simulink model "im_foc_models_decouple"  (R2022b)
settings: Solver=VariableStepAuto  StartTime=0.0  StopTime=1  FixedStep=0.001  RelTol=1e-3
undefined symbols (not defined in the file): B, c, J, k, K1, K2, K3, K4, K5, K6, Lm, Lr, pole
libraries: slpidlib x5
settings Model: Creator=jack  LastModifiedBy=jackyeh

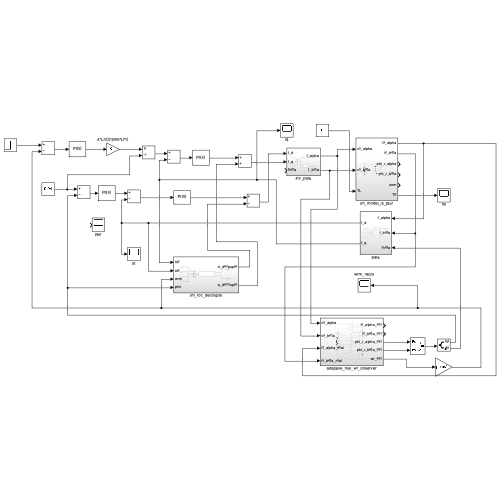
[thumbnail: Simulink's stored preview of the top-level diagram]
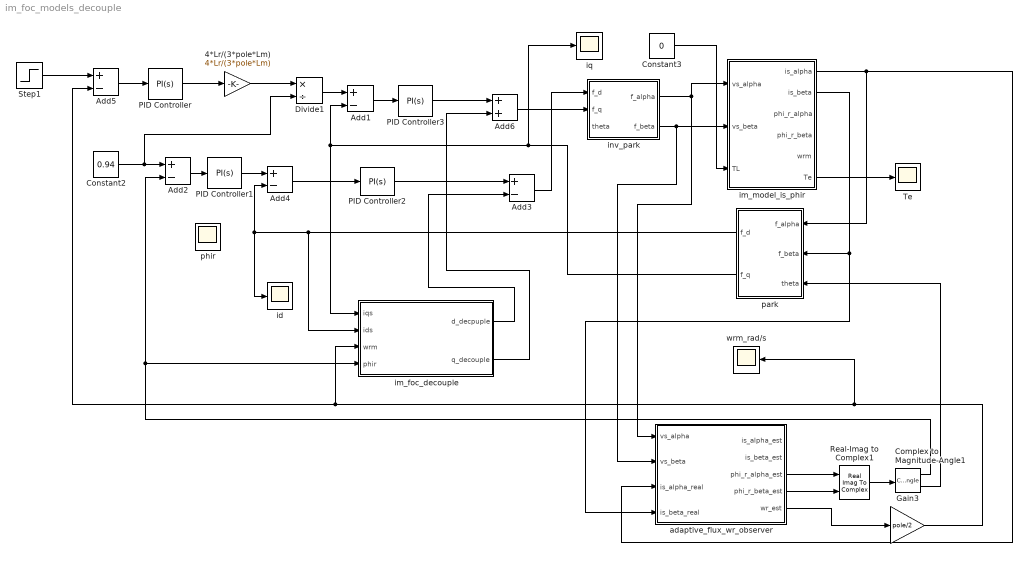
== system im_foc_models_decouple ==
  4*Lr/(3*pole*Lm) : Gain  Gain=4*Lr/(3*pole*Lm)
  Add{1..5} (5 alike) : Sum  Inputs=+-
  Add6 : Sum
  Complex to Magnitude-Angle1 : ComplexToMagnitudeAngle
  Constant2 : Constant  Value=0.94
  Constant3 : Constant  Value=0
  Divide1 : Product  Inputs=*/
  Gain3 : Gain  Gain=pole/2
  PID Controller : slpidlib/PID Controller  Controller=PI  Form=Parallel  TimeDomain=Continuous-time  UseExternalTs=off  SampleTime=-1  IntegratorMethod=Forward Euler  FilterMethod=Forward Euler  ControllerParametersSource=internal  P=1.65  I=0.41  UseKiTs=off  D=0  N=100  UseFilter=on  TunerSelectOption=Transfer Function Based (PID Tuner App)  InitialConditionSource=internal  InitialConditionForIntegrator=0  InitialConditionForFilter=0  DifferentiatorICPrevScaledInput=0  ExternalReset=none  TrackingMode=off  Kt=1  LimitOutput=off  SatLimitsSource=internal  UpperSaturationLimit=inf  LowerSaturationLimit=-inf  LinearizeAsGain=on  AntiWindupMode=none  Kb=1  LimitIntegrator=off  UpperIntegratorSaturationLimit=inf  LowerIntegratorSaturationLimit=-inf  POutMin=[]  POutMax=[]  IOutMin=[]  IOutMax=[]  DOutMin=[]  DOutMax=[]  NOutMin=[]  NOutMax=[]  SumOutMin=[]  SumOutMax=[]  SaturationOutMin=[]  SaturationOutMax=[]  PParamMin=[]  PParamMax=[]  IParamMin=[]  IParamMax=[]  DParamMin=[]  DParamMax=[]  NParamMin=[]  NParamMax=[]  KbParamMin=[]  KbParamMax=[]  KtParamMin=[]  KtParamMax=[]  KbOutMin=[]  KbOutMax=[]  KtOutMin=[]  KtOutMax=[]  IntegratorOutMin=[]  IntegratorOutMax=[]  FilterOutMin=[]  FilterOutMax=[]  SumI1OutMin=[]  SumI1OutMax=[]  SumI2OutMin=[]  SumI2OutMax=[]  SumI3OutMin=[]  SumI3OutMax=[]  SumI4OutMin=[]  SumI4OutMax=[]  SumDOutMin=[]  SumDOutMax=[]  DifferentiatorOutMin=[]  DifferentiatorOutMax=[]  FilterDiffOutCoefMin=[]  FilterDiffOutCoefMax=[]  ReciprocalOutMin=[]  ReciprocalOutMax=[]  SumDenOutMin=[]  SumDenOutMax=[]  SumNumOutMin=[]  SumNumOutMax=[]  DivideOutMin=[]  DivideOutMax=[]  UdiffTsProdOutMin=[]  UdiffTsProdOutMax=[]  NTsProdOutMin=[]  NTsProdOutMax=[]  UintegralTsProdOutMin=[]  UintegralTsProdOutMax=[]  UngainTsProdOutMin=[]  UngainTsProdOutMax=[]  ClampingZeroOutDataTypeStr=Inherit: Inherit via back propagation  ClampingZeroOutMin=[]  ClampingZeroOutMax=[]  FilterDenConstantOutDataTypeStr=Inherit: Inherit via back propagation  FilterDenConstantOutMin=[]  FilterDenConstantOutMax=[]  PCopyOutDataTypeStr=Inherit: Inherit via back propagation  PCopyOutMin=[]  PCopyOutMax=[]  NCopyOutDataTypeStr=Inherit: Inherit via back propagation  NCopyOutMin=[]  NCopyOutMax=[]  IntegratorContinuousStateAttributes=''  IntegratorStateMustResolveToSignalObject=off  IntegratorRTWStateStorageClass=Auto  FilterContinuousStateAttributes=''  FilterStateMustResolveToSignalObject=off  FilterRTWStateStorageClass=Auto  ParallelPVariant=InternalParameters  IdealPVariant=Disabled  IVariant=InternalParameters  DVariant=Disabled  IntegratorVariant=Continuous  SatVariant=Disabled  AWVariant=Passthrough  PCopyVariant=Disabled  TRVariant=Disabled  FdbkBlocksVariant=Forward  IdealPFdbkVariant=Disabled  SatFdbkVariant=Disabled  DerivativeFilterVariant=Disabled  NVariant=Disabled  NCopyVariant=Disabled_SignalSpec  FilterICVariant=Disabled  IntegratorICVariant=InternalICs  ExternalResetVariant=Disabled  TRSumVariant=Passthrough  SumFdbkVariant=Disabled  SumVariant=Sum_PI  TsampFilterVariant=InternalTs  TsampNgainVariant=Passthrough  TsampIntegralVariant=Passthrough  ExternalSaturationOutDataTypeStr=Inherit: Same as second input
  PID Controller1 : slpidlib/PID Controller  Controller=PI  Form=Parallel  TimeDomain=Continuous-time  UseExternalTs=off  SampleTime=-1  IntegratorMethod=Forward Euler  FilterMethod=Forward Euler  ControllerParametersSource=internal  P=86.38  I=609.76  UseKiTs=off  D=0  N=100  UseFilter=on  TunerSelectOption=Transfer Function Based (PID Tuner App)  InitialConditionSource=internal  InitialConditionForIntegrator=0  InitialConditionForFilter=0  DifferentiatorICPrevScaledInput=0  ExternalReset=none  TrackingMode=off  Kt=1  LimitOutput=off  SatLimitsSource=internal  UpperSaturationLimit=inf  LowerSaturationLimit=-inf  LinearizeAsGain=on  AntiWindupMode=none  Kb=1  LimitIntegrator=off  UpperIntegratorSaturationLimit=inf  LowerIntegratorSaturationLimit=-inf  POutMin=[]  POutMax=[]  IOutMin=[]  IOutMax=[]  DOutMin=[]  DOutMax=[]  NOutMin=[]  NOutMax=[]  SumOutMin=[]  SumOutMax=[]  SaturationOutMin=[]  SaturationOutMax=[]  PParamMin=[]  PParamMax=[]  IParamMin=[]  IParamMax=[]  DParamMin=[]  DParamMax=[]  NParamMin=[]  NParamMax=[]  KbParamMin=[]  KbParamMax=[]  KtParamMin=[]  KtParamMax=[]  KbOutMin=[]  KbOutMax=[]  KtOutMin=[]  KtOutMax=[]  IntegratorOutMin=[]  IntegratorOutMax=[]  FilterOutMin=[]  FilterOutMax=[]  SumI1OutMin=[]  SumI1OutMax=[]  SumI2OutMin=[]  SumI2OutMax=[]  SumI3OutMin=[]  SumI3OutMax=[]  SumI4OutMin=[]  SumI4OutMax=[]  SumDOutMin=[]  SumDOutMax=[]  DifferentiatorOutMin=[]  DifferentiatorOutMax=[]  FilterDiffOutCoefMin=[]  FilterDiffOutCoefMax=[]  ReciprocalOutMin=[]  ReciprocalOutMax=[]  SumDenOutMin=[]  SumDenOutMax=[]  SumNumOutMin=[]  SumNumOutMax=[]  DivideOutMin=[]  DivideOutMax=[]  UdiffTsProdOutMin=[]  UdiffTsProdOutMax=[]  NTsProdOutMin=[]  NTsProdOutMax=[]  UintegralTsProdOutMin=[]  UintegralTsProdOutMax=[]  UngainTsProdOutMin=[]  UngainTsProdOutMax=[]  ClampingZeroOutDataTypeStr=Inherit: Inherit via back propagation  ClampingZeroOutMin=[]  ClampingZeroOutMax=[]  FilterDenConstantOutDataTypeStr=Inherit: Inherit via back propagation  FilterDenConstantOutMin=[]  FilterDenConstantOutMax=[]  PCopyOutDataTypeStr=Inherit: Inherit via back propagation  PCopyOutMin=[]  PCopyOutMax=[]  NCopyOutDataTypeStr=Inherit: Inherit via back propagation  NCopyOutMin=[]  NCopyOutMax=[]  IntegratorContinuousStateAttributes=''  IntegratorStateMustResolveToSignalObject=off  IntegratorRTWStateStorageClass=Auto  FilterContinuousStateAttributes=''  FilterStateMustResolveToSignalObject=off  FilterRTWStateStorageClass=Auto  ParallelPVariant=InternalParameters  IdealPVariant=Disabled  IVariant=InternalParameters  DVariant=Disabled  IntegratorVariant=Continuous  SatVariant=Disabled  AWVariant=Passthrough  PCopyVariant=Disabled  TRVariant=Disabled  FdbkBlocksVariant=Forward  IdealPFdbkVariant=Disabled  SatFdbkVariant=Disabled  DerivativeFilterVariant=Disabled  NVariant=Disabled  NCopyVariant=Disabled_SignalSpec  FilterICVariant=Disabled  IntegratorICVariant=InternalICs  ExternalResetVariant=Disabled  TRSumVariant=Passthrough  SumFdbkVariant=Disabled  SumVariant=Sum_PI  TsampFilterVariant=InternalTs  TsampNgainVariant=Passthrough  TsampIntegralVariant=Passthrough  ExternalSaturationOutDataTypeStr=Inherit: Same as second input
  PID Controller2 : slpidlib/PID Controller  Controller=PI  Form=Parallel  TimeDomain=Continuous-time  UseExternalTs=off  SampleTime=-1  IntegratorMethod=Forward Euler  FilterMethod=Forward Euler  ControllerParametersSource=internal  P=2.95  I=679.2  UseKiTs=off  D=0  N=100  UseFilter=on  TunerSelectOption=Transfer Function Based (PID Tuner App)  InitialConditionSource=internal  InitialConditionForIntegrator=0  InitialConditionForFilter=0  DifferentiatorICPrevScaledInput=0  ExternalReset=none  TrackingMode=off  Kt=1  LimitOutput=off  SatLimitsSource=internal  UpperSaturationLimit=inf  LowerSaturationLimit=-inf  LinearizeAsGain=on  AntiWindupMode=none  Kb=1  LimitIntegrator=off  UpperIntegratorSaturationLimit=inf  LowerIntegratorSaturationLimit=-inf  POutMin=[]  POutMax=[]  IOutMin=[]  IOutMax=[]  DOutMin=[]  DOutMax=[]  NOutMin=[]  NOutMax=[]  SumOutMin=[]  SumOutMax=[]  SaturationOutMin=[]  SaturationOutMax=[]  PParamMin=[]  PParamMax=[]  IParamMin=[]  IParamMax=[]  DParamMin=[]  DParamMax=[]  NParamMin=[]  NParamMax=[]  KbParamMin=[]  KbParamMax=[]  KtParamMin=[]  KtParamMax=[]  KbOutMin=[]  KbOutMax=[]  KtOutMin=[]  KtOutMax=[]  IntegratorOutMin=[]  IntegratorOutMax=[]  FilterOutMin=[]  FilterOutMax=[]  SumI1OutMin=[]  SumI1OutMax=[]  SumI2OutMin=[]  SumI2OutMax=[]  SumI3OutMin=[]  SumI3OutMax=[]  SumI4OutMin=[]  SumI4OutMax=[]  SumDOutMin=[]  SumDOutMax=[]  DifferentiatorOutMin=[]  DifferentiatorOutMax=[]  FilterDiffOutCoefMin=[]  FilterDiffOutCoefMax=[]  ReciprocalOutMin=[]  ReciprocalOutMax=[]  SumDenOutMin=[]  SumDenOutMax=[]  SumNumOutMin=[]  SumNumOutMax=[]  DivideOutMin=[]  DivideOutMax=[]  UdiffTsProdOutMin=[]  UdiffTsProdOutMax=[]  NTsProdOutMin=[]  NTsProdOutMax=[]  UintegralTsProdOutMin=[]  UintegralTsProdOutMax=[]  UngainTsProdOutMin=[]  UngainTsProdOutMax=[]  ClampingZeroOutDataTypeStr=Inherit: Inherit via back propagation  ClampingZeroOutMin=[]  ClampingZeroOutMax=[]  FilterDenConstantOutDataTypeStr=Inherit: Inherit via back propagation  FilterDenConstantOutMin=[]  FilterDenConstantOutMax=[]  PCopyOutDataTypeStr=Inherit: Inherit via back propagation  PCopyOutMin=[]  PCopyOutMax=[]  NCopyOutDataTypeStr=Inherit: Inherit via back propagation  NCopyOutMin=[]  NCopyOutMax=[]  IntegratorContinuousStateAttributes=''  IntegratorStateMustResolveToSignalObject=off  IntegratorRTWStateStorageClass=Auto  FilterContinuousStateAttributes=''  FilterStateMustResolveToSignalObject=off  FilterRTWStateStorageClass=Auto  ParallelPVariant=InternalParameters  IdealPVariant=Disabled  IVariant=InternalParameters  DVariant=Disabled  IntegratorVariant=Continuous  SatVariant=Disabled  AWVariant=Passthrough  PCopyVariant=Disabled  TRVariant=Disabled  FdbkBlocksVariant=Forward  IdealPFdbkVariant=Disabled  SatFdbkVariant=Disabled  DerivativeFilterVariant=Disabled  NVariant=Disabled  NCopyVariant=Disabled_SignalSpec  FilterICVariant=Disabled  IntegratorICVariant=InternalICs  ExternalResetVariant=Disabled  TRSumVariant=Passthrough  SumFdbkVariant=Disabled  SumVariant=Sum_PI  TsampFilterVariant=InternalTs  TsampNgainVariant=Passthrough  TsampIntegralVariant=Passthrough  ExternalSaturationOutDataTypeStr=Inherit: Same as second input
  PID Controller3 : slpidlib/PID Controller  Controller=PI  Form=Parallel  TimeDomain=Continuous-time  UseExternalTs=off  SampleTime=-1  IntegratorMethod=Forward Euler  FilterMethod=Forward Euler  ControllerParametersSource=internal  P=2.95  I=400  UseKiTs=off  D=0  N=100  UseFilter=on  TunerSelectOption=Transfer Function Based (PID Tuner App)  InitialConditionSource=internal  InitialConditionForIntegrator=0  InitialConditionForFilter=0  DifferentiatorICPrevScaledInput=0  ExternalReset=none  TrackingMode=off  Kt=1  LimitOutput=off  SatLimitsSource=internal  UpperSaturationLimit=inf  LowerSaturationLimit=-inf  LinearizeAsGain=on  AntiWindupMode=none  Kb=1  LimitIntegrator=off  UpperIntegratorSaturationLimit=inf  LowerIntegratorSaturationLimit=-inf  POutMin=[]  POutMax=[]  IOutMin=[]  IOutMax=[]  DOutMin=[]  DOutMax=[]  NOutMin=[]  NOutMax=[]  SumOutMin=[]  SumOutMax=[]  SaturationOutMin=[]  SaturationOutMax=[]  PParamMin=[]  PParamMax=[]  IParamMin=[]  IParamMax=[]  DParamMin=[]  DParamMax=[]  NParamMin=[]  NParamMax=[]  KbParamMin=[]  KbParamMax=[]  KtParamMin=[]  KtParamMax=[]  KbOutMin=[]  KbOutMax=[]  KtOutMin=[]  KtOutMax=[]  IntegratorOutMin=[]  IntegratorOutMax=[]  FilterOutMin=[]  FilterOutMax=[]  SumI1OutMin=[]  SumI1OutMax=[]  SumI2OutMin=[]  SumI2OutMax=[]  SumI3OutMin=[]  SumI3OutMax=[]  SumI4OutMin=[]  SumI4OutMax=[]  SumDOutMin=[]  SumDOutMax=[]  DifferentiatorOutMin=[]  DifferentiatorOutMax=[]  FilterDiffOutCoefMin=[]  FilterDiffOutCoefMax=[]  ReciprocalOutMin=[]  ReciprocalOutMax=[]  SumDenOutMin=[]  SumDenOutMax=[]  SumNumOutMin=[]  SumNumOutMax=[]  DivideOutMin=[]  DivideOutMax=[]  UdiffTsProdOutMin=[]  UdiffTsProdOutMax=[]  NTsProdOutMin=[]  NTsProdOutMax=[]  UintegralTsProdOutMin=[]  UintegralTsProdOutMax=[]  UngainTsProdOutMin=[]  UngainTsProdOutMax=[]  ClampingZeroOutDataTypeStr=Inherit: Inherit via back propagation  ClampingZeroOutMin=[]  ClampingZeroOutMax=[]  FilterDenConstantOutDataTypeStr=Inherit: Inherit via back propagation  FilterDenConstantOutMin=[]  FilterDenConstantOutMax=[]  PCopyOutDataTypeStr=Inherit: Inherit via back propagation  PCopyOutMin=[]  PCopyOutMax=[]  NCopyOutDataTypeStr=Inherit: Inherit via back propagation  NCopyOutMin=[]  NCopyOutMax=[]  IntegratorContinuousStateAttributes=''  IntegratorStateMustResolveToSignalObject=off  IntegratorRTWStateStorageClass=Auto  FilterContinuousStateAttributes=''  FilterStateMustResolveToSignalObject=off  FilterRTWStateStorageClass=Auto  ParallelPVariant=InternalParameters  IdealPVariant=Disabled  IVariant=InternalParameters  DVariant=Disabled  IntegratorVariant=Continuous  SatVariant=Disabled  AWVariant=Passthrough  PCopyVariant=Disabled  TRVariant=Disabled  FdbkBlocksVariant=Forward  IdealPFdbkVariant=Disabled  SatFdbkVariant=Disabled  DerivativeFilterVariant=Disabled  NVariant=Disabled  NCopyVariant=Disabled_SignalSpec  FilterICVariant=Disabled  IntegratorICVariant=InternalICs  ExternalResetVariant=Disabled  TRSumVariant=Passthrough  SumFdbkVariant=Disabled  SumVariant=Sum_PI  TsampFilterVariant=InternalTs  TsampNgainVariant=Passthrough  TsampIntegralVariant=Passthrough  ExternalSaturationOutDataTypeStr=Inherit: Same as second input
  Real-Imag to Complex1 : RealImagToComplex
  Step1 : Step  Time=0  After=100  SampleTime=0
  Te : Scope
  adaptive_flux_wr_observer : Subsystem
  id : Scope
  im_foc_decouple : Subsystem
  im_model_is_phir : Subsystem
  inv_park : Subsystem
  iq : Scope
  park : Subsystem
  phir : Scope
  wrm_rad/s : Scope
  wires:
  PID Controller/1 -> 4*Lr/(3*pole*Lm)/1
  4*Lr/(3*pole*Lm)/1 -> Divide1/1
  Constant2/1 -> Divide1/2, Add2/1
  Divide1/1 -> Add1/1
  Add1/1 -> PID Controller3/1
  Add2/1 -> PID Controller1/1
  PID Controller1/1 -> Add4/1
  Add4/1 -> PID Controller2/1
  Add5/1 -> PID Controller/1
  Add6/1 -> inv_park/2(f_q)
  inv_park/1(f_alpha) -> im_model_is_phir/1(vs_alpha), adaptive_flux_wr_observer/1(vs_alpha)
  inv_park/2(f_beta) -> im_model_is_phir/2(vs_beta), adaptive_flux_wr_observer/2(vs_beta)
  Constant3/1 -> im_model_is_phir/3(TL)
  im_model_is_phir/1(is_alpha) -> adaptive_flux_wr_observer/3(is_alpha_real), park/1(f_alpha)
  im_model_is_phir/2(is_beta) -> adaptive_flux_wr_observer/4(is_beta_real), park/2(f_beta)
  park/2(f_q) -> im_foc_decouple/1(iqs), Add1/2, iq/1
  park/1(f_d) -> im_foc_decouple/2(ids), Add4/2, id/1
  Add3/1 -> inv_park/1(f_d)
  im_model_is_phir/6(Te) -> Te/1
  PID Controller2/1 -> Add3/1
  im_foc_decouple/1(d_decpuple) -> Add3/2
  PID Controller3/1 -> Add6/1
  im_foc_decouple/2(q_decouple) -> Add6/2
  Step1/1 -> Add5/1
  adaptive_flux_wr_observer/3(phi_r_alpha_est) -> Real-Imag to Complex1/1
  adaptive_flux_wr_observer/4(phi_r_beta_est) -> Real-Imag to Complex1/2
  Real-Imag to Complex1/1 -> Complex to Magnitude-Angle1/1
  Complex to Magnitude-Angle1/2 -> park/3(theta)
  Complex to Magnitude-Angle1/1 -> Add2/2, im_foc_decouple/4(phir)
  adaptive_flux_wr_observer/5(wr_est) -> Gain3/1
  Gain3/1 -> wrm_rad/s/1, im_foc_decouple/3(wrm), Add5/2

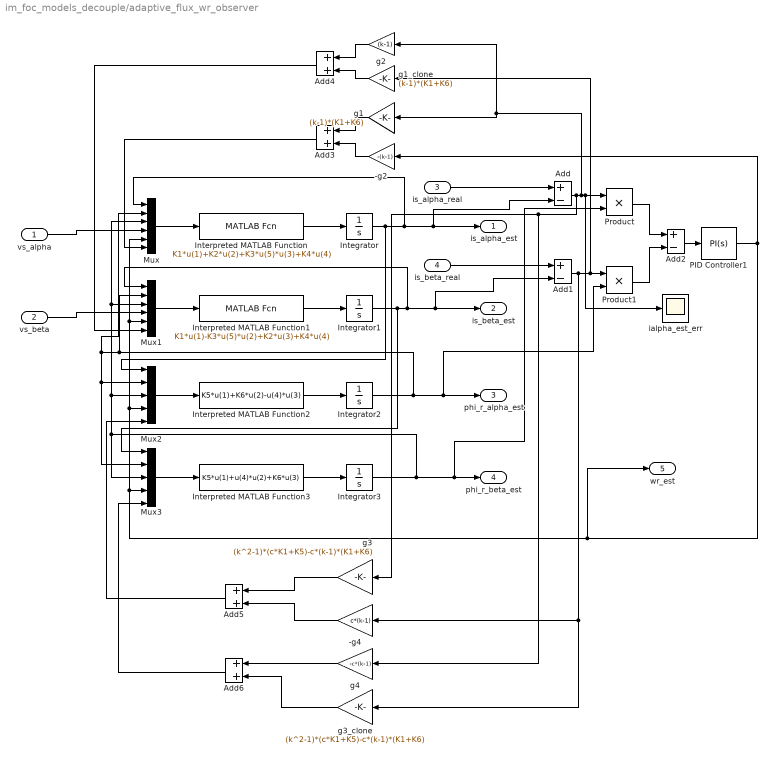
== system im_foc_models_decouple/adaptive_flux_wr_observer ==
  vs_alpha : Inport
  vs_beta : Inport  Port=2
  is_alpha_real : Inport  Port=3
  is_beta_real : Inport  Port=4
  -g2 : Gain  Gain=-(k-1)
  -g4 : Gain  Gain=c*(k-1)
  Add : Sum  Inputs=+-
  Add1 : Sum  Inputs=+-
  Add2 : Sum  Inputs=+-
  Add{3..6} (4 alike) : Sum
  Integrator{,1..3} (4 alike) : Integrator
  Interpreted MATLAB Function : MATLABFcn  MATLABFcn=K1*u(1)+K2*u(2)+K3*u(5)*u(3)+K4*u(4)
  Interpreted MATLAB Function1 : MATLABFcn  MATLABFcn=K1*u(1)-K3*u(5)*u(2)+K2*u(3)+K4*u(4)
  Interpreted MATLAB Function2 : MATLABFcn  MATLABFcn=K5*u(1)+K6*u(2)-u(4)*u(3)
  Interpreted MATLAB Function3 : MATLABFcn  MATLABFcn=K5*u(1)+u(4)*u(2)+K6*u(3)
  Mux : Mux  Inputs=6
  Mux1 : Mux  Inputs=6
  Mux2 : Mux  Inputs=5
  Mux3 : Mux  Inputs=5
  PID Controller1 : slpidlib/PID Controller  Controller=PI  Form=Parallel  TimeDomain=Continuous-time  UseExternalTs=off  SampleTime=-1  IntegratorMethod=Forward Euler  FilterMethod=Forward Euler  ControllerParametersSource=internal  P=542  I=3829  UseKiTs=off  D=0  N=100  UseFilter=on  TunerSelectOption=Transfer Function Based (PID Tuner App)  InitialConditionSource=internal  InitialConditionForIntegrator=0  InitialConditionForFilter=0  DifferentiatorICPrevScaledInput=0  ExternalReset=none  TrackingMode=off  Kt=1  LimitOutput=off  SatLimitsSource=internal  UpperSaturationLimit=inf  LowerSaturationLimit=-inf  LinearizeAsGain=on  AntiWindupMode=none  Kb=1  LimitIntegrator=off  UpperIntegratorSaturationLimit=inf  LowerIntegratorSaturationLimit=-inf  POutMin=[]  POutMax=[]  IOutMin=[]  IOutMax=[]  DOutMin=[]  DOutMax=[]  NOutMin=[]  NOutMax=[]  SumOutMin=[]  SumOutMax=[]  SaturationOutMin=[]  SaturationOutMax=[]  PParamMin=[]  PParamMax=[]  IParamMin=[]  IParamMax=[]  DParamMin=[]  DParamMax=[]  NParamMin=[]  NParamMax=[]  KbParamMin=[]  KbParamMax=[]  KtParamMin=[]  KtParamMax=[]  KbOutMin=[]  KbOutMax=[]  KtOutMin=[]  KtOutMax=[]  IntegratorOutMin=[]  IntegratorOutMax=[]  FilterOutMin=[]  FilterOutMax=[]  SumI1OutMin=[]  SumI1OutMax=[]  SumI2OutMin=[]  SumI2OutMax=[]  SumI3OutMin=[]  SumI3OutMax=[]  SumI4OutMin=[]  SumI4OutMax=[]  SumDOutMin=[]  SumDOutMax=[]  DifferentiatorOutMin=[]  DifferentiatorOutMax=[]  FilterDiffOutCoefMin=[]  FilterDiffOutCoefMax=[]  ReciprocalOutMin=[]  ReciprocalOutMax=[]  SumDenOutMin=[]  SumDenOutMax=[]  SumNumOutMin=[]  SumNumOutMax=[]  DivideOutMin=[]  DivideOutMax=[]  UdiffTsProdOutMin=[]  UdiffTsProdOutMax=[]  NTsProdOutMin=[]  NTsProdOutMax=[]  UintegralTsProdOutMin=[]  UintegralTsProdOutMax=[]  UngainTsProdOutMin=[]  UngainTsProdOutMax=[]  ClampingZeroOutDataTypeStr=Inherit: Inherit via back propagation  ClampingZeroOutMin=[]  ClampingZeroOutMax=[]  FilterDenConstantOutDataTypeStr=Inherit: Inherit via back propagation  FilterDenConstantOutMin=[]  FilterDenConstantOutMax=[]  PCopyOutDataTypeStr=Inherit: Inherit via back propagation  PCopyOutMin=[]  PCopyOutMax=[]  NCopyOutDataTypeStr=Inherit: Inherit via back propagation  NCopyOutMin=[]  NCopyOutMax=[]  IntegratorContinuousStateAttributes=''  IntegratorStateMustResolveToSignalObject=off  IntegratorRTWStateStorageClass=Auto  FilterContinuousStateAttributes=''  FilterStateMustResolveToSignalObject=off  FilterRTWStateStorageClass=Auto  ParallelPVariant=InternalParameters  IdealPVariant=Disabled  IVariant=InternalParameters  DVariant=Disabled  IntegratorVariant=Continuous  SatVariant=Disabled  AWVariant=Passthrough  PCopyVariant=Disabled  TRVariant=Disabled  FdbkBlocksVariant=Forward  IdealPFdbkVariant=Disabled  SatFdbkVariant=Disabled  DerivativeFilterVariant=Disabled  NVariant=Disabled  NCopyVariant=Disabled_SignalSpec  FilterICVariant=Disabled  IntegratorICVariant=InternalICs  ExternalResetVariant=Disabled  TRSumVariant=Passthrough  SumFdbkVariant=Disabled  SumVariant=Sum_PI  TsampFilterVariant=InternalTs  TsampNgainVariant=Passthrough  TsampIntegralVariant=Passthrough  ExternalSaturationOutDataTypeStr=Inherit: Same as second input
  Product : Product
  Product1 : Product
  g1 : Gain  Gain=(k-1)*(K1+K6)
  g1_clone : Gain  Gain=(k-1)*(K1+K6)
  g2 : Gain  Gain=(k-1)
  g3 : Gain  Gain=(k^2-1)*(c*K1+K5)-c*(k-1)*(K1+K6)
  g3_clone : Gain  Gain=(k^2-1)*(c*K1+K5)-c*(k-1)*(K1+K6)
  g4 : Gain  Gain=-c*(k-1)
  ialpha_est_err : Scope
  is_alpha_est : Outport
  is_beta_est : Outport  Port=2
  phi_r_alpha_est : Outport  Port=3
  phi_r_beta_est : Outport  Port=4
  wr_est : Outport  Port=5
  wires:
  Add3/1 -> Mux/6
  is_alpha_real/1 -> Add/1
  Mux1/1 -> Interpreted MATLAB Function1/1
  Interpreted MATLAB Function1/1 -> Integrator1/1
  Mux/1 -> Interpreted MATLAB Function/1
  Product1/1 -> Add2/2
  Integrator3/1 -> phi_r_beta_est/1, Product/2, Mux3/3, Mux2/3, Mux/3, Mux1/3
  vs_beta/1 -> Mux1/4
  Add5/1 -> Mux2/5
  Add/1 -> g4/1, g3/1, g2/1, g1/1, ialpha_est_err/1, Product/1
  is_beta_real/1 -> Add1/1
  Add4/1 -> Mux1/6
  g3/1 -> Add5/1
  g1_clone/1 -> Add4/2
  Integrator/1 -> Mux2/1, is_alpha_est/1, Add/2, Mux/1
  g1/1 -> Add3/1
  Interpreted MATLAB Function3/1 -> Integrator3/1
  g4/1 -> Add6/1
  Interpreted MATLAB Function/1 -> Integrator/1
  vs_alpha/1 -> Mux/4
  Add2/1 -> PID Controller1/1
  PID Controller1/1 -> wr_est/1, Mux3/4, Mux2/4, Mux1/5, Mux/5, -g2/1
  -g4/1 -> Add5/2
  Mux3/1 -> Interpreted MATLAB Function3/1
  g2/1 -> Add4/1
  Add6/1 -> Mux3/5
  Interpreted MATLAB Function2/1 -> Integrator2/1
  Integrator2/1 -> phi_r_alpha_est/1, Product1/2, Mux1/2, Mux/2, Mux3/2, Mux2/2
  Mux2/1 -> Interpreted MATLAB Function2/1
  -g2/1 -> Add3/2
  Product/1 -> Add2/1
  Integrator1/1 -> Mux3/1, is_beta_est/1, Add1/2, Mux1/1
  Add1/1 -> -g4/1, g3_clone/1, g1_clone/1, Product1/1
  g3_clone/1 -> Add6/2

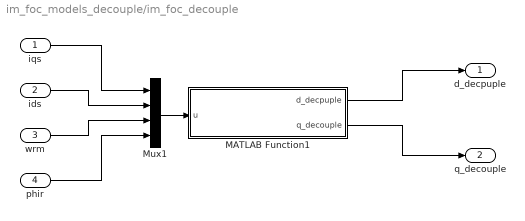
== system im_foc_models_decouple/im_foc_decouple ==
  iqs : Inport
  ids : Inport  Port=2
  wrm : Inport  Port=3
  phir : Inport  Port=4
  MATLAB Function1 : MATLAB Function  TreatAsAtomicUnit=on
  Mux1 : Mux
  d_decpuple : Outport
  q_decouple : Outport  Port=2
  wires:
  iqs/1 -> Mux1/1
  ids/1 -> Mux1/2
  wrm/1 -> Mux1/3
  Mux1/1 -> MATLAB Function1/1(u)
  MATLAB Function1/1(d_decpuple) -> d_decpuple/1
  MATLAB Function1/2(q_decouple) -> q_decouple/1
  phir/1 -> Mux1/4

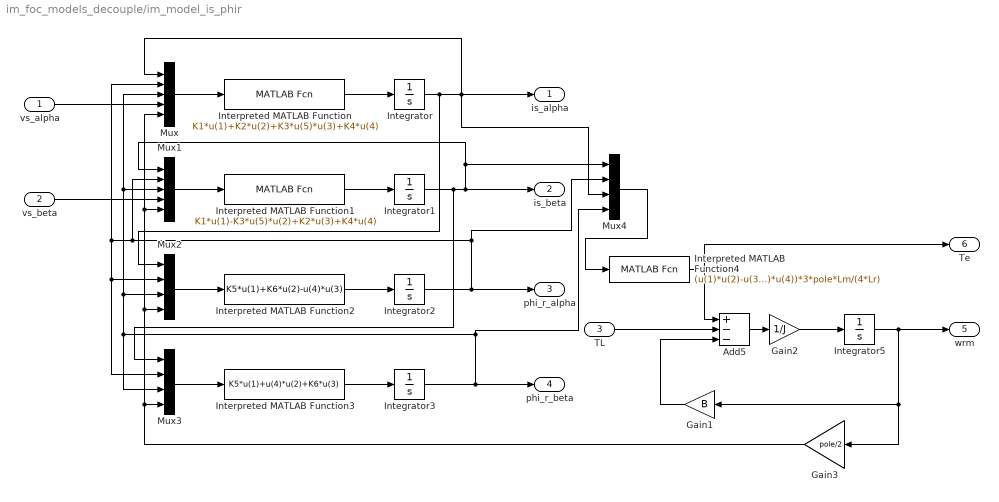
== system im_foc_models_decouple/im_model_is_phir ==
  vs_alpha : Inport
  vs_beta : Inport  Port=2
  TL : Inport  Port=3
  Add5 : Sum  Inputs=+--
  Gain1 : Gain  Gain=B
  Gain2 : Gain  Gain=1/J
  Gain3 : Gain  Gain=pole/2
  Integrator{,1..3,5} (5 alike) : Integrator
  Interpreted MATLAB Function : MATLABFcn  MATLABFcn=K1*u(1)+K2*u(2)+K3*u(5)*u(3)+K4*u(4)
  Interpreted MATLAB Function1 : MATLABFcn  MATLABFcn=K1*u(1)-K3*u(5)*u(2)+K2*u(3)+K4*u(4)
  Interpreted MATLAB Function2 : MATLABFcn  MATLABFcn=K5*u(1)+K6*u(2)-u(4)*u(3)
  Interpreted MATLAB Function3 : MATLABFcn  MATLABFcn=K5*u(1)+u(4)*u(2)+K6*u(3)
  Interpreted MATLAB Function4 : MATLABFcn  MATLABFcn=(u(1)*u(2)-u(3)*u(4))*3*pole*Lm/(4*Lr)
  Mux : Mux  Inputs=5
  Mux1 : Mux  Inputs=5
  Mux2 : Mux
  Mux3 : Mux
  Mux4 : Mux
  is_alpha : Outport
  is_beta : Outport  Port=2
  phi_r_alpha : Outport  Port=3
  phi_r_beta : Outport  Port=4
  wrm : Outport  Port=5
  Te : Outport  Port=6
  wires:
  Add5/1 -> Gain2/1
  Interpreted MATLAB Function2/1 -> Integrator2/1
  vs_beta/1 -> Mux1/4
  vs_alpha/1 -> Mux/4
  Mux3/1 -> Interpreted MATLAB Function3/1
  Interpreted MATLAB Function1/1 -> Integrator1/1
  Mux4/1 -> Interpreted MATLAB Function4/1
  Integrator1/1 -> Mux3/1, is_beta/1, Mux1/1, Mux4/1
  Gain1/1 -> Add5/3
  TL/1 -> Add5/2
  Interpreted MATLAB Function4/1 -> Te/1, Add5/1
  Integrator5/1 -> wrm/1, Gain1/1, Gain3/1
  Integrator2/1 -> phi_r_alpha/1, Mux4/2, Mux1/2, Mux/2, Mux3/2, Mux2/2
  Integrator3/1 -> phi_r_beta/1, Mux4/4, Mux3/3, Mux2/3, Mux/3, Mux1/3
  Mux1/1 -> Interpreted MATLAB Function1/1
  Interpreted MATLAB Function3/1 -> Integrator3/1
  Mux2/1 -> Interpreted MATLAB Function2/1
  Mux/1 -> Interpreted MATLAB Function/1
  Gain2/1 -> Integrator5/1
  Interpreted MATLAB Function/1 -> Integrator/1
  Integrator/1 -> Mux2/1, is_alpha/1, Mux4/3, Mux/1
  Gain3/1 -> Mux3/4, Mux2/4, Mux1/5, Mux/5

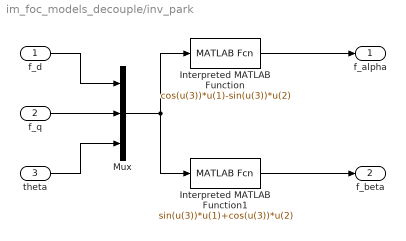
== system im_foc_models_decouple/inv_park ==
  f_d : Inport
  f_q : Inport  Port=2
  theta : Inport  Port=3
  Interpreted MATLAB Function : MATLABFcn  MATLABFcn=cos(u(3))*u(1)-sin(u(3))*u(2)
  Interpreted MATLAB Function1 : MATLABFcn  MATLABFcn=sin(u(3))*u(1)+cos(u(3))*u(2)
  Mux : Mux  Inputs=3
  f_alpha : Outport
  f_beta : Outport  Port=2
  wires:
  Interpreted MATLAB Function/1 -> f_alpha/1
  f_d/1 -> Mux/1
  Mux/1 -> Interpreted MATLAB Function1/1, Interpreted MATLAB Function/1
  Interpreted MATLAB Function1/1 -> f_beta/1
  theta/1 -> Mux/3
  f_q/1 -> Mux/2

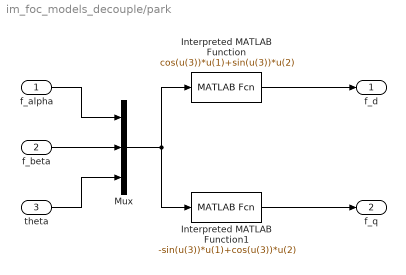
== system im_foc_models_decouple/park ==
  f_alpha : Inport
  f_beta : Inport  Port=2
  theta : Inport  Port=3
  Interpreted MATLAB Function : MATLABFcn  MATLABFcn=cos(u(3))*u(1)+sin(u(3))*u(2)
  Interpreted MATLAB Function1 : MATLABFcn  MATLABFcn=-sin(u(3))*u(1)+cos(u(3))*u(2)
  Mux : Mux  Inputs=3
  f_d : Outport
  f_q : Outport  Port=2
  wires:
  Interpreted MATLAB Function/1 -> f_d/1
  f_alpha/1 -> Mux/1
  Mux/1 -> Interpreted MATLAB Function1/1, Interpreted MATLAB Function/1
  Interpreted MATLAB Function1/1 -> f_q/1
  theta/1 -> Mux/3
  f_beta/1 -> Mux/2

== matlab function im_foc_models_decouple/im_foc_decouple/MATLAB Function1 ==
  data: u input; d_decpuple output; q_decouple output
function [d_decpuple, q_decouple] = decouple(u)
    Rr = 0.6;
    Lr = 0.085;
    Ls = 0.085;
    Lm = 0.082;
    sigma = 1 - Lm^2/(Ls*Lr);
    w = Ls*Lr - Lm^2;
    Lsigma = w/Lr;
    Tr = Lr/Rr;
    pole = 4;
    wslip = (u(1)*Rr)/(u(2)*Lr+1e-8);
    we = wslip + u(3)*pole/2;
    d_decpuple = Lsigma*(we*u(1) + (1-sigma)/(sigma*Lm*Tr)*u(4));
    q_decouple = Lsigma*(we*u(2) + (1-sigma)/(sigma*Lm)*we*u(4));
